simulink model "lab2"  (R2022a)
settings: Solver=ode4  StartTime=0.0  StopTime=5  FixedStep=0.002  RelTol=1e-3  EnableMultiTasking=on
libraries: quarc_library x2
settings Model: ExtModeTrigDuration=10000  Creator=20wds  LastModifiedBy=20wds
settings SolverCC: AlgebraicLoopSolver=TrustRegion  PositivePriorityOrder=on
settings DataIOCC: ReturnWorkspaceOutputs=off
settings DebuggingCC: UnconnectedInputMsg=warning  UnconnectedOutputMsg=warning  UnconnectedLineMsg=warning  SFMachineParentedDataDiag=warning  ArithmeticOperatorsInVariantConditions=warning
settings SFSimCC: SimUseLocalCustomCode=off  CustomCodeUndefinedFunction=UseInterfaceOnly
settings RTWCC: Description=QUARC Win64 Target Using Toolchain  SystemTargetFile=quarc_win64.tlc  TemplateMakefile=quarc_default_tmf  RTWUseLocalCustomCode=off  Toolchain=QUARC win64 | nmake (64-bit Windows)  BuildConfiguration=Faster Runs
settings CodeAppCC: StateflowObjectComments=on
settings STFCustomTargetCC: TargetLangStandard=C99 (ISO)  ConcurrentExecutionCompliant=on  UseToolchainInfoCompliant=on  SystemTargetFile=quarc_win64.tlc
settings GRTTargetCC: ParMdlRefBuildCompliant=off  CompOptLevelCompliant=off  CombineOutputUpdateFcns=off  MatFileLogging=off  CPPClassGenCompliant=off  GRTInterface=on  ExtMode=on  ExtModeMexFile=quarc_comm
settings ConfigComp: CovMetricSettings=dswe

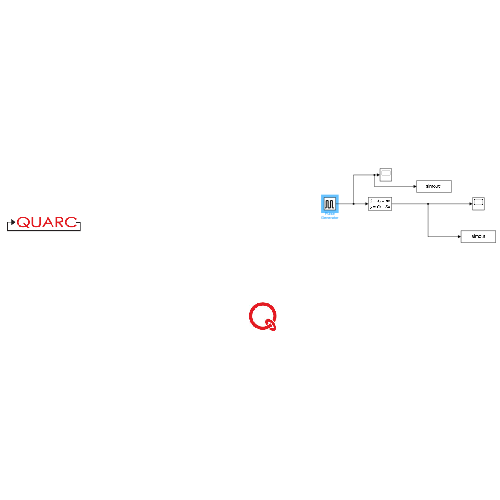
[thumbnail: Simulink's stored preview of the top-level diagram]
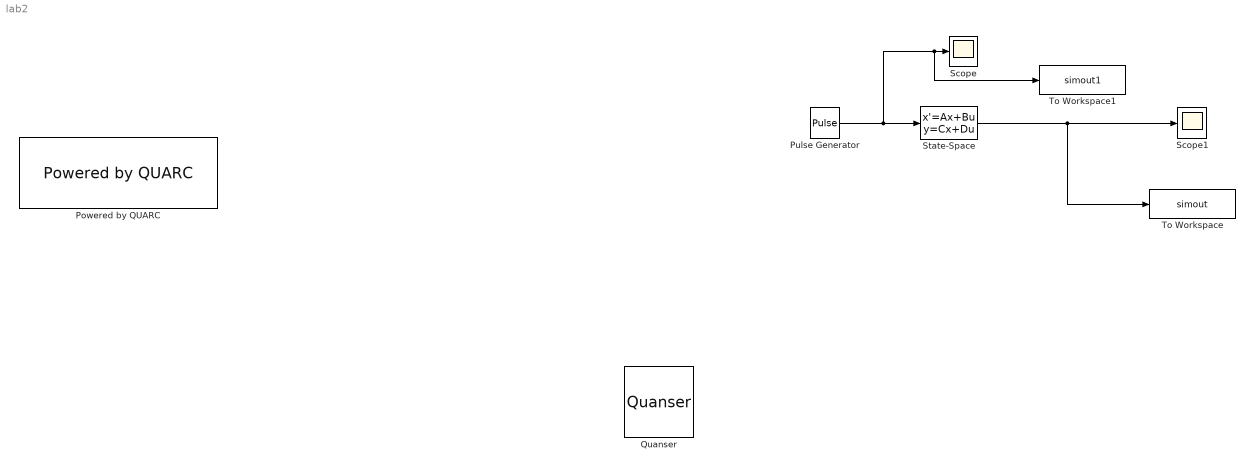
== system lab2 ==
  Powered by QUARC : quarc_library/Logos/Powered by QUARC
  Pulse Generator : DiscretePulseGenerator  PulseType=Time based  Amplitude=10  Period=10  PulseWidth=0.1/10*100
  Quanser : quarc_library/Logos/Quanser
  Scope : Scope
  Scope1 : Scope
  State-Space : StateSpace  A=[0 1; 0 -1/0.028]  B=[0; 250]  C=[1 0; 0 1]  D=[0; 0]  InitialCondition=0
  To Workspace : ToWorkspace  VariableName=simout  SaveFormat=Structure With Time  SampleTime=-1
  To Workspace1 : ToWorkspace  VariableName=simout1  SaveFormat=Structure With Time  SampleTime=-1
  wires:
  Pulse Generator/1 -> To Workspace1/1, Scope/1, State-Space/1
  State-Space/1 -> To Workspace/1, Scope1/1
